simulink model "COSTEP"  (R2024b)
settings: Solver=FixedStepAuto  StartTime=0.0  StopTime=25  FixedStep=1/3600  RelTol=1e-3
model workspace (MAT data in the model file):
  AD : Simulink.Parameter (value not decoded)
  AG : Simulink.Parameter (value not decoded)
  AH : Simulink.Parameter (value not decoded)
  AV : Simulink.Parameter (value not decoded)
  AVP : Simulink.Parameter (value not decoded)
  BCHL : Simulink.Parameter (value not decoded)
  BCHV : Simulink.Parameter (value not decoded)
  BD : Simulink.Parameter (value not decoded)
  BDIST : Simulink.Parameter (value not decoded)
  BG : Simulink.Parameter (value not decoded)
  BH : Simulink.Parameter (value not decoded)
  BVP : Simulink.Parameter (value not decoded)
  CD : Simulink.Parameter (value not decoded)
  CDIST : Simulink.Parameter (value not decoded)
  CG : Simulink.Parameter (value not decoded)
  CH : Simulink.Parameter (value not decoded)
  CVP : Simulink.Parameter (value not decoded)
  DDIST : Simulink.Parameter (value not decoded)
  DIST_CONST : Simulink.Parameter (value not decoded)
  ISV : Simulink.Parameter (value not decoded)
  TLAST : Simulink.Parameter (value not decoded)
  TNEXT : Simulink.Parameter (value not decoded)
  XMW : Simulink.Parameter (value not decoded)
  XNS : Simulink.Parameter (value not decoded)
  XNS2 : Simulink.Parameter (value not decoded)
  XNS3 : Simulink.Parameter (value not decoded)
  XNSADD : Simulink.Parameter (value not decoded)
  XNSE : Simulink.Parameter (value not decoded)
symbols that are objects in the model workspace (value not decoded): AD, AG, AH, AV, AVP, BD, BG, BH, BVP, CD, CG, CH, CVP, XMW, XNS, XNS2, XNS3, XNSE
undefined symbols (not defined in the file or in its folder): magnitude, msgbox, SETPT, XMEAS, XMV
libraries: mylib x381, dspindex x31
(part 10 of 12)

== system COSTEP/Stream Measurements/Subsystem6/Condenser product stream/Subsystem/TST(8a) Temperature of Stream °C  ==
  HST : Inport  PortDimensions=1
  XLR : Inport  Port=2  PortDimensions=8
  ITY : Inport  Port=3
  "AG(I) Coefficient A to determine Enthalpy MBtu/lb·°F " : Constant  Value=AG
  "AH(I) Coefficient A to determine Enthalpy MBtu/lb·°F " : Constant  Value=AH
  AV(I) Coefficient AV to determine Enthalpy MBtu/lb : Constant  Value=AV
  BG(I) Coefficient B to determine Enthalpy MBtu/lb·°F² : Constant  Value=BG
  BH(I) Coefficient B to determine Enthalpy MBtu/lb·°F² : Constant  Value=BH
  CG(I) Coefficient C to determine Enthalpy MBtu/lb·°F³ : Constant  Value=CG
  CH(I) Coefficient C to determine Enthalpy MBtu/lb·°F³ : Constant  Value=CH
  Delay : Delay  DelayLength=1  InitialCondition=0
  MATLAB Function : MATLAB Function  TreatAsAtomicUnit=on
  "XMW(I) Molecular weight of components lb/lb-mol " : Constant  Value=XMW
  TST(8a) : Outport  PortDimensions=1  VectorParamsAs1DForOutWhenUnconnected=off
  wires:
  MATLAB Function/1(TST) -> Delay/1, TST(8a)/1
  Delay/1 -> MATLAB Function/12("TST ")
  "AG(I) Coefficient A to determine Enthalpy MBtu/lb·°F "/1 -> MATLAB Function/4(AG)
  AV(I) Coefficient AV to determine Enthalpy MBtu/lb/1 -> MATLAB Function/7(AV)
  HST/1 -> MATLAB Function/10(HST)
  CH(I) Coefficient C to determine Enthalpy MBtu/lb·°F³/1 -> MATLAB Function/3(CH)
  ITY/1 -> MATLAB Function/11(ITY)
  "XMW(I) Molecular weight of components lb/lb-mol "/1 -> MATLAB Function/8(XMW)
  XLR/1 -> MATLAB Function/9(XLR)
  "AH(I) Coefficient A to determine Enthalpy MBtu/lb·°F "/1 -> MATLAB Function/1(AH)
  CG(I) Coefficient C to determine Enthalpy MBtu/lb·°F³/1 -> MATLAB Function/6(CG)
  BH(I) Coefficient B to determine Enthalpy MBtu/lb·°F²/1 -> MATLAB Function/2(BH)
  BG(I) Coefficient B to determine Enthalpy MBtu/lb·°F²/1 -> MATLAB Function/5(BG)

== system COSTEP/Stream Measurements/Subsystem6/D feed stream/Composition measurement mol%/Subsystem ==
  XST : Inport
  XMNSE : Inport  Port=2
  Bus Selector : BusSelector  OutputSignals=XMNSEB,XMNSED
  Process Noise I=23-1 : mylib/Process Noise I=23-36  SystemSampleTime=-1  VariantActivationTime=update diagram  AllowFlexibleInterface=on  Latency=0  AutoFrameSizeCalculation=off
  Process Noise I=23-3 : mylib/Process Noise I=23-36  SystemSampleTime=-1  VariantActivationTime=update diagram  AllowFlexibleInterface=on  Latency=0  AutoFrameSizeCalculation=off
  Subsystem : Subsystem
  SMEASXB(2) : Outport  VectorParamsAs1DForOutWhenUnconnected=off
  SMEASXD(2) : Outport  Port=2  VectorParamsAs1DForOutWhenUnconnected=off
  wires:
  Process Noise I=23-1/1 -> SMEASXB(2)/1
  Bus Selector/1 -> Process Noise I=23-1/2  "<XMNSEB>"
  Process Noise I=23-3/1 -> SMEASXD(2)/1
  Bus Selector/2 -> Process Noise I=23-3/2  "<XMNSED>"
  XST/1 -> Subsystem/1(XST)
  Subsystem/1(XCMPB) -> Process Noise I=23-1/1
  Subsystem/2(XCMPD) -> Process Noise I=23-3/1
  XMNSE/1 -> Bus Selector/1

== system COSTEP/Stream Measurements/Subsystem6/E feed stream/Composition measurement mol%/Subsystem ==
  XST : Inport
  XMNSE : Inport  Port=2
  Bus Selector : BusSelector  OutputSignals=XMNSEE,XMNSEF
  Process Noise I=23-4 : mylib/Process Noise I=23-36  SystemSampleTime=-1  VariantActivationTime=update diagram  AllowFlexibleInterface=on  Latency=0  AutoFrameSizeCalculation=off
  Process Noise I=23-5 : mylib/Process Noise I=23-36  SystemSampleTime=-1  VariantActivationTime=update diagram  AllowFlexibleInterface=on  Latency=0  AutoFrameSizeCalculation=off
  Subsystem : Subsystem
  SMEASXE(3) : Outport  VectorParamsAs1DForOutWhenUnconnected=off
  SMEASXF(3) : Outport  Port=2  VectorParamsAs1DForOutWhenUnconnected=off
  wires:
  Process Noise I=23-4/1 -> SMEASXE(3)/1
  Process Noise I=23-5/1 -> SMEASXF(3)/1
  Bus Selector/2 -> Process Noise I=23-5/2  "<XMNSEF>"
  Bus Selector/1 -> Process Noise I=23-4/2  "<XMNSEE>"
  XST/1 -> Subsystem/1(XST)
  Subsystem/1("XCMPE ") -> Process Noise I=23-4/1
  Subsystem/2("XCMPF ") -> Process Noise I=23-5/1
  XMNSE/1 -> Bus Selector/1

== system COSTEP/Stream Measurements/Subsystem6/Product stream/Composition measurement mol%/Subsystem ==
  XST : Inport
  XMNSE : Inport  Port=2
  Bus Selector : BusSelector  OutputSignals=XMNSEA,XMNSEB,XMNSEC
  Process Noise I=23-1 : mylib/Process Noise I=23-36  SystemSampleTime=-1  VariantActivationTime=update diagram  AllowFlexibleInterface=on  Latency=0  AutoFrameSizeCalculation=off
  Process Noise I=23-2 : mylib/Process Noise I=23-36  SystemSampleTime=-1  VariantActivationTime=update diagram  AllowFlexibleInterface=on  Latency=0  AutoFrameSizeCalculation=off
  Process Noise I=23-36 : mylib/Process Noise I=23-36  SystemSampleTime=-1  VariantActivationTime=update diagram  AllowFlexibleInterface=on  Latency=0  AutoFrameSizeCalculation=off
  Subsystem : Subsystem
  SMEASXA : Outport  VectorParamsAs1DForOutWhenUnconnected=off
  SMEASXB : Outport  Port=2  VectorParamsAs1DForOutWhenUnconnected=off
  SMEASXC : Outport  Port=3  VectorParamsAs1DForOutWhenUnconnected=off
  wires:
  Process Noise I=23-36/1 -> SMEASXA/1
  Process Noise I=23-1/1 -> SMEASXB/1
  Bus Selector/2 -> Process Noise I=23-1/2  "<XMNSEB>"
  Process Noise I=23-2/1 -> SMEASXC/1
  Bus Selector/3 -> Process Noise I=23-2/2  "<XMNSEC>"
  Bus Selector/1 -> Process Noise I=23-36/2  "<XMNSEA>"
  XST/1 -> Subsystem/1(XST)
  Subsystem/1(XCMPA) -> Process Noise I=23-36/1
  Subsystem/2(XCMPB) -> Process Noise I=23-1/1
  Subsystem/3(XCMPC) -> Process Noise I=23-2/1
  XMNSE/1 -> Bus Selector/1

== system COSTEP/Stream Measurements/Subsystem6/Product stream/Composition measurement mol%/Subsystem1 ==
  XST : Inport
  XMNSE3 : Inport  Port=2
  Bus Selector : BusSelector  OutputSignals=XMNSED,XMNSEE,XMNSEF,XMNSEG,XMNSEH
  Process Noise I=37-{1..4,41} (5 alike) : mylib/Process Noise I=37-41  SystemSampleTime=-1  VariantActivationTime=update diagram  AllowFlexibleInterface=on  Latency=0  AutoFrameSizeCalculation=off
  Subsystem : Subsystem
  SMEASXD : Outport  VectorParamsAs1DForOutWhenUnconnected=off
  SMEASXE : Outport  Port=2  VectorParamsAs1DForOutWhenUnconnected=off
  SMEASXF : Outport  Port=3  VectorParamsAs1DForOutWhenUnconnected=off
  SMEASXG : Outport  Port=4  VectorParamsAs1DForOutWhenUnconnected=off
  SMEASXH : Outport  Port=5  VectorParamsAs1DForOutWhenUnconnected=off
  wires:
  Process Noise I=37-41/1 -> SMEASXD/1
  Bus Selector/1 -> Process Noise I=37-41/2  "<XMNSED>"
  Process Noise I=37-1/1 -> SMEASXE/1
  Bus Selector/2 -> Process Noise I=37-1/2  "<XMNSEE>"
  Process Noise I=37-2/1 -> SMEASXF/1
  Bus Selector/3 -> Process Noise I=37-2/2  "<XMNSEF>"
  Process Noise I=37-3/1 -> SMEASXG/1
  Bus Selector/4 -> Process Noise I=37-3/2  "<XMNSEG>"
  Process Noise I=37-4/1 -> SMEASXH/1
  Bus Selector/5 -> Process Noise I=37-4/2  "<XMNSEH>"
  XST/1 -> Subsystem/1(XST)
  Subsystem/1(XCMPD) -> Process Noise I=37-41/1
  Subsystem/2("XCMPE ") -> Process Noise I=37-1/1
  Subsystem/3("XCMPF ") -> Process Noise I=37-2/1
  Subsystem/4(XCMPG) -> Process Noise I=37-3/1
  Subsystem/5("XCMPH ") -> Process Noise I=37-4/1
  XMNSE3/1 -> Bus Selector/1

== system COSTEP/Stream Measurements/Subsystem6/Product stream/Flow measurement in kg//h/XMWS Molecular weight of Stream lb//lb-mol ==
  XST : Inport
  Product : Product
  Sum of Elements : Sum  Inputs=+
  "XMW(I) Molecular weight of components lb/lb-mol " : Constant  Value=XMW
  XMWS : Outport  VectorParamsAs1DForOutWhenUnconnected=off
  wires:
  Sum of Elements/1 -> XMWS/1
  Product/1 -> Sum of Elements/1
  XST/1 -> Product/1
  "XMW(I) Molecular weight of components lb/lb-mol "/1 -> Product/2

== system COSTEP/Stream Measurements/Subsystem6/Purge stream/Flow measurement in kg//h/XMWS Molecular weight of Stream lb//lb-mol ==
  XST : Inport
  Product : Product
  Sum of Elements : Sum  Inputs=+
  "XMW(I) Molecular weight of components lb/lb-mol " : Constant  Value=XMW
  XMWS : Outport  VectorParamsAs1DForOutWhenUnconnected=off
  wires:
  Sum of Elements/1 -> XMWS/1
  Product/1 -> Sum of Elements/1
  XST/1 -> Product/1
  "XMW(I) Molecular weight of components lb/lb-mol "/1 -> Product/2

== system COSTEP/Stream Measurements/Subsystem6/Reactor feed stream/Composition measurement mol%/Subsystem ==
  XST : Inport
  XMNSE : Inport  Port=2
  XMEAS : Inport  Port=3
  Bus Selector : BusSelector  OutputSignals=XMNSEG,XMNSEH
  Bus Selector1 : BusSelector  OutputSignals=XMEAS(23),XMEAS(24),XMEAS(25),XMEAS(26),XMEAS(27),XMEAS(28)
  Process Noise I=23-6 : mylib/Process Noise I=23-36  SystemSampleTime=-1  VariantActivationTime=update diagram  AllowFlexibleInterface=on  Latency=0  AutoFrameSizeCalculation=off
  Process Noise I=23-7 : mylib/Process Noise I=23-36  SystemSampleTime=-1  VariantActivationTime=update diagram  AllowFlexibleInterface=on  Latency=0  AutoFrameSizeCalculation=off
  Subsystem : Subsystem
  SMEASXA : Outport  VectorParamsAs1DForOutWhenUnconnected=off
  SMEASXB : Outport  Port=2  VectorParamsAs1DForOutWhenUnconnected=off
  SMEASXC : Outport  Port=3  VectorParamsAs1DForOutWhenUnconnected=off
  SMEASXD : Outport  Port=4  VectorParamsAs1DForOutWhenUnconnected=off
  SMEASXE : Outport  Port=5  VectorParamsAs1DForOutWhenUnconnected=off
  SMEASXF : Outport  Port=6  VectorParamsAs1DForOutWhenUnconnected=off
  SMEASXG : Outport  Port=7  VectorParamsAs1DForOutWhenUnconnected=off
  SMEASXH : Outport  Port=8  VectorParamsAs1DForOutWhenUnconnected=off
  wires:
  Bus Selector1/1 -> SMEASXA/1  "<XMEAS(23)>"
  Bus Selector1/2 -> SMEASXB/1  "<XMEAS(24)>"
  Bus Selector1/3 -> SMEASXC/1  "<XMEAS(25)>"
  Bus Selector1/4 -> SMEASXD/1  "<XMEAS(26)>"
  Bus Selector1/5 -> SMEASXE/1  "<XMEAS(27)>"
  Bus Selector1/6 -> SMEASXF/1  "<XMEAS(28)>"
  Process Noise I=23-6/1 -> SMEASXG/1
  Process Noise I=23-7/1 -> SMEASXH/1
  Bus Selector/1 -> Process Noise I=23-6/2  "<XMNSEG>"
  Bus Selector/2 -> Process Noise I=23-7/2  "<XMNSEH>"
  XST/1 -> Subsystem/1(XST)
  Subsystem/1(XCMPG) -> Process Noise I=23-6/1
  Subsystem/2("XCMPH ") -> Process Noise I=23-7/1
  XMNSE/1 -> Bus Selector/1
  XMEAS/1 -> Bus Selector1/1

== system COSTEP/Stream Measurements/Subsystem6/Reactor feed stream/Flow measurement in kg//h/XMWS Molecular weight of Stream lb//lb-mol ==
  XST : Inport
  Product : Product
  Sum of Elements : Sum  Inputs=+
  "XMW(I) Molecular weight of components lb/lb-mol " : Constant  Value=XMW
  XMWS : Outport  VectorParamsAs1DForOutWhenUnconnected=off
  wires:
  Sum of Elements/1 -> XMWS/1
  Product/1 -> Sum of Elements/1
  XST/1 -> Product/1
  "XMW(I) Molecular weight of components lb/lb-mol "/1 -> Product/2

== system COSTEP/Stream Measurements/Subsystem6/Reactor product stream/Composition measurement mol%/Subsystem ==
  XST : Inport
  XMNSE : Inport  Port=2
  Bus Selector : BusSelector  OutputSignals=XMNSEA,XMNSEB,XMNSEC,XMNSED,XMNSEE,XMNSEF,XMNSEG,XMNSEH
  Process Noise I=23-{1..7,36} (8 alike) : mylib/Process Noise I=23-36  SystemSampleTime=-1  VariantActivationTime=update diagram  AllowFlexibleInterface=on  Latency=0  AutoFrameSizeCalculation=off
  Subsystem : Subsystem
  SMEASXA(7) : Outport  VectorParamsAs1DForOutWhenUnconnected=off
  SMEASXB(7) : Outport  Port=2  VectorParamsAs1DForOutWhenUnconnected=off
  SMEASXC(7) : Outport  Port=3  VectorParamsAs1DForOutWhenUnconnected=off
  SMEASXD(7) : Outport  Port=4  VectorParamsAs1DForOutWhenUnconnected=off
  SMEASXE(7) : Outport  Port=5  VectorParamsAs1DForOutWhenUnconnected=off
  SMEASXF(7) : Outport  Port=6  VectorParamsAs1DForOutWhenUnconnected=off
  SMEASXG(7) : Outport  Port=7  VectorParamsAs1DForOutWhenUnconnected=off
  SMEASXH(7) : Outport  Port=8  VectorParamsAs1DForOutWhenUnconnected=off
  wires:
  Process Noise I=23-36/1 -> SMEASXA(7)/1
  Process Noise I=23-1/1 -> SMEASXB(7)/1
  Bus Selector/2 -> Process Noise I=23-1/2  "<XMNSEB>"
  Process Noise I=23-2/1 -> SMEASXC(7)/1
  Process Noise I=23-3/1 -> SMEASXD(7)/1
  Process Noise I=23-4/1 -> SMEASXE(7)/1
  Process Noise I=23-5/1 -> SMEASXF(7)/1
  Process Noise I=23-6/1 -> SMEASXG(7)/1
  Process Noise I=23-7/1 -> SMEASXH(7)/1
  Bus Selector/7 -> Process Noise I=23-6/2  "<XMNSEG>"
  Bus Selector/8 -> Process Noise I=23-7/2  "<XMNSEH>"
  Bus Selector/6 -> Process Noise I=23-5/2  "<XMNSEF>"
  Bus Selector/5 -> Process Noise I=23-4/2  "<XMNSEE>"
  Bus Selector/4 -> Process Noise I=23-3/2  "<XMNSED>"
  Bus Selector/3 -> Process Noise I=23-2/2  "<XMNSEC>"
  Bus Selector/1 -> Process Noise I=23-36/2  "<XMNSEA>"
  XST/1 -> Subsystem/1(XST)
  Subsystem/1(XCMPA) -> Process Noise I=23-36/1
  Subsystem/2(XCMPB) -> Process Noise I=23-1/1
  Subsystem/3(XCMPC) -> Process Noise I=23-2/1
  Subsystem/4(XCMPD) -> Process Noise I=23-3/1
  Subsystem/5("XCMPE ") -> Process Noise I=23-4/1
  Subsystem/6("XCMPF ") -> Process Noise I=23-5/1
  Subsystem/7(XCMPG) -> Process Noise I=23-6/1
  Subsystem/8("XCMPH ") -> Process Noise I=23-7/1
  XMNSE/1 -> Bus Selector/1

== system COSTEP/Stream Measurements/Subsystem6/Reactor product stream/Flow measurement in kg//h/XMWS Molecular weight of Stream lb//lb-mol ==
  XST : Inport
  Product : Product
  Sum of Elements : Sum  Inputs=+
  "XMW(I) Molecular weight of components lb/lb-mol " : Constant  Value=XMW
  XMWS : Outport  VectorParamsAs1DForOutWhenUnconnected=off
  wires:
  Sum of Elements/1 -> XMWS/1
  Product/1 -> Sum of Elements/1
  XST/1 -> Product/1
  "XMW(I) Molecular weight of components lb/lb-mol "/1 -> Product/2

== system COSTEP/Stream Measurements/Subsystem6/Separator product stream/Composition measurement mol%/Subsystem ==
  XST : Inport
  XMNSE : Inport  Port=2
  Bus Selector : BusSelector  OutputSignals=XMNSEA,XMNSEB,XMNSEC,XMNSED,XMNSEE,XMNSEF,XMNSEG,XMNSEH
  Process Noise I=23-{1..7,36} (8 alike) : mylib/Process Noise I=23-36  SystemSampleTime=-1  VariantActivationTime=update diagram  AllowFlexibleInterface=on  Latency=0  AutoFrameSizeCalculation=off
  Subsystem : Subsystem
  SMEASXA : Outport  VectorParamsAs1DForOutWhenUnconnected=off
  SMEASXB : Outport  Port=2  VectorParamsAs1DForOutWhenUnconnected=off
  SMEASXC : Outport  Port=3  VectorParamsAs1DForOutWhenUnconnected=off
  SMEASXD : Outport  Port=4  VectorParamsAs1DForOutWhenUnconnected=off
  SMEASXE : Outport  Port=5  VectorParamsAs1DForOutWhenUnconnected=off
  SMEASXF : Outport  Port=6  VectorParamsAs1DForOutWhenUnconnected=off
  SMEASXG : Outport  Port=7  VectorParamsAs1DForOutWhenUnconnected=off
  SMEASXH : Outport  Port=8  VectorParamsAs1DForOutWhenUnconnected=off
  wires:
  Process Noise I=23-36/1 -> SMEASXA/1
  Process Noise I=23-1/1 -> SMEASXB/1
  Bus Selector/2 -> Process Noise I=23-1/2  "<XMNSEB>"
  Process Noise I=23-2/1 -> SMEASXC/1
  Process Noise I=23-3/1 -> SMEASXD/1
  Process Noise I=23-4/1 -> SMEASXE/1
  Process Noise I=23-5/1 -> SMEASXF/1
  Process Noise I=23-6/1 -> SMEASXG/1
  Process Noise I=23-7/1 -> SMEASXH/1
  Bus Selector/7 -> Process Noise I=23-6/2  "<XMNSEG>"
  Bus Selector/8 -> Process Noise I=23-7/2  "<XMNSEH>"
  Bus Selector/6 -> Process Noise I=23-5/2  "<XMNSEF>"
  Bus Selector/5 -> Process Noise I=23-4/2  "<XMNSEE>"
  Bus Selector/4 -> Process Noise I=23-3/2  "<XMNSED>"
  Bus Selector/3 -> Process Noise I=23-2/2  "<XMNSEC>"
  Bus Selector/1 -> Process Noise I=23-36/2  "<XMNSEA>"
  XST/1 -> Subsystem/1(XST)
  Subsystem/1(XCMPA) -> Process Noise I=23-36/1
  Subsystem/2(XCMPB) -> Process Noise I=23-1/1
  Subsystem/3(XCMPC) -> Process Noise I=23-2/1
  Subsystem/4(XCMPD) -> Process Noise I=23-3/1
  Subsystem/5("XCMPE ") -> Process Noise I=23-4/1
  Subsystem/6("XCMPF ") -> Process Noise I=23-5/1
  Subsystem/7(XCMPG) -> Process Noise I=23-6/1
  Subsystem/8("XCMPH ") -> Process Noise I=23-7/1
  XMNSE/1 -> Bus Selector/1

== system COSTEP/Stream Measurements/Subsystem6/Separator product stream/Flow measurement in kg//h/Subsystem ==
  XST : Inport
  XMEAS : Inport  Port=2
  " " : Constant  Value=35.3145
  "  " : Constant  Value=0.359
  Convert from lb/h to kg/h : Constant  Value=0.454
  Product : Product  Inputs=3
  XMWS Molecular weight of Stream lb/lb-mol : Subsystem
  lb-mol/h : Product  Inputs=**/
  SMEAS F : Outport
  wires:
  lb-mol/h/1 -> Product/2
  " "/1 -> lb-mol/h/2
  XST/1 -> XMWS Molecular weight of Stream lb/lb-mol/1(XST)
  "  "/1 -> lb-mol/h/3
  Product/1 -> SMEAS F/1
  Convert from lb/h to kg/h/1 -> Product/3
  XMWS Molecular weight of Stream lb/lb-mol/1(XMWS) -> Product/1
  XMEAS/1 -> lb-mol/h/1

== system COSTEP/Stream Measurements/Subsystem6/Separator product stream/Flow measurement in kg//h/Subsystem1 ==
  XST : Inport
  XMEAS : Inport  Port=2
  " " : Constant  Value=35.3145
  "  " : Constant  Value=0.359
  Convert from lb/h to kg/h : Constant  Value=0.454
  Product : Product  Inputs=3
  XMWS Molecular weight of Stream lb/lb-mol : Subsystem
  lb-mol/h : Product  Inputs=**/
  SMEAS F : Outport
  wires:
  lb-mol/h/1 -> Product/2
  " "/1 -> lb-mol/h/2
  XST/1 -> XMWS Molecular weight of Stream lb/lb-mol/1(XST)
  "  "/1 -> lb-mol/h/3
  Product/1 -> SMEAS F/1
  Convert from lb/h to kg/h/1 -> Product/3
  XMWS Molecular weight of Stream lb/lb-mol/1(XMWS) -> Product/1
  XMEAS/1 -> lb-mol/h/1

== system COSTEP/Stream Measurements/Subsystem6/Separator recycle stream (after compressor)/Composition measurement mol%/Subsystem ==
  XST : Inport
  XMNSE : Inport  Port=2
  Bus Selector : BusSelector  OutputSignals=XMNSEA,XMNSEB,XMNSEC,XMNSED,XMNSEE,XMNSEF,XMNSEG,XMNSEH
  Process Noise I=23-{1..7,36} (8 alike) : mylib/Process Noise I=23-36  SystemSampleTime=-1  VariantActivationTime=update diagram  AllowFlexibleInterface=on  Latency=0  AutoFrameSizeCalculation=off
  Subsystem : Subsystem
  SMEASXA : Outport  VectorParamsAs1DForOutWhenUnconnected=off
  SMEASXB : Outport  Port=2  VectorParamsAs1DForOutWhenUnconnected=off
  SMEASXC : Outport  Port=3  VectorParamsAs1DForOutWhenUnconnected=off
  SMEASXD : Outport  Port=4  VectorParamsAs1DForOutWhenUnconnected=off
  SMEASXE : Outport  Port=5  VectorParamsAs1DForOutWhenUnconnected=off
  SMEASXF : Outport  Port=6  VectorParamsAs1DForOutWhenUnconnected=off
  SMEASXG : Outport  Port=7  VectorParamsAs1DForOutWhenUnconnected=off
  SMEASXH : Outport  Port=8  VectorParamsAs1DForOutWhenUnconnected=off
  wires:
  Process Noise I=23-36/1 -> SMEASXA/1
  Process Noise I=23-1/1 -> SMEASXB/1
  Bus Selector/2 -> Process Noise I=23-1/2  "<XMNSEB>"
  Process Noise I=23-2/1 -> SMEASXC/1
  Process Noise I=23-3/1 -> SMEASXD/1
  Process Noise I=23-4/1 -> SMEASXE/1
  Process Noise I=23-5/1 -> SMEASXF/1
  Process Noise I=23-6/1 -> SMEASXG/1
  Process Noise I=23-7/1 -> SMEASXH/1
  Bus Selector/7 -> Process Noise I=23-6/2  "<XMNSEG>"
  Bus Selector/8 -> Process Noise I=23-7/2  "<XMNSEH>"
  Bus Selector/6 -> Process Noise I=23-5/2  "<XMNSEF>"
  Bus Selector/5 -> Process Noise I=23-4/2  "<XMNSEE>"
  Bus Selector/4 -> Process Noise I=23-3/2  "<XMNSED>"
  Bus Selector/3 -> Process Noise I=23-2/2  "<XMNSEC>"
  Bus Selector/1 -> Process Noise I=23-36/2  "<XMNSEA>"
  XST/1 -> Subsystem/1(XST)
  Subsystem/1(XCMPA) -> Process Noise I=23-36/1
  Subsystem/2(XCMPB) -> Process Noise I=23-1/1
  Subsystem/3(XCMPC) -> Process Noise I=23-2/1
  Subsystem/4(XCMPD) -> Process Noise I=23-3/1
  Subsystem/5("XCMPE ") -> Process Noise I=23-4/1
  Subsystem/6("XCMPF ") -> Process Noise I=23-5/1
  Subsystem/7(XCMPG) -> Process Noise I=23-6/1
  Subsystem/8("XCMPH ") -> Process Noise I=23-7/1
  XMNSE/1 -> Bus Selector/1

== system COSTEP/Stream Measurements/Subsystem6/Separator recycle stream (after compressor)/Flow measurement in kg//h/XMWS Molecular weight of Stream lb//lb-mol ==
  XST : Inport
  Product : Product
  Sum of Elements : Sum  Inputs=+
  "XMW(I) Molecular weight of components lb/lb-mol " : Constant  Value=XMW
  XMWS : Outport  VectorParamsAs1DForOutWhenUnconnected=off
  wires:
  Sum of Elements/1 -> XMWS/1
  Product/1 -> Sum of Elements/1
  XST/1 -> Product/1
  "XMW(I) Molecular weight of components lb/lb-mol "/1 -> Product/2

== system COSTEP/Stream Measurements/Subsystem6/Separator recycle stream (after compressor)/Temperature measurement in C/TST(9) Temperature of Stream °C  ==
  HST : Inport  PortDimensions=1
  XLR : Inport  Port=2  PortDimensions=8
  ITY : Inport  Port=3
  "AG(I) Coefficient A to determine Enthalpy MBtu/lb·°F " : Constant  Value=AG
  "AH(I) Coefficient A to determine Enthalpy MBtu/lb·°F " : Constant  Value=AH
  AV(I) Coefficient AV to determine Enthalpy MBtu/lb : Constant  Value=AV
  BG(I) Coefficient B to determine Enthalpy MBtu/lb·°F² : Constant  Value=BG
  BH(I) Coefficient B to determine Enthalpy MBtu/lb·°F² : Constant  Value=BH
  CG(I) Coefficient C to determine Enthalpy MBtu/lb·°F³ : Constant  Value=CG
  CH(I) Coefficient C to determine Enthalpy MBtu/lb·°F³ : Constant  Value=CH
  Delay : Delay  DelayLength=1  InitialCondition=0
  MATLAB Function : MATLAB Function  TreatAsAtomicUnit=on
  "XMW(I) Molecular weight of components lb/lb-mol " : Constant  Value=XMW
  TST(9) : Outport  PortDimensions=1  VectorParamsAs1DForOutWhenUnconnected=off
  wires:
  MATLAB Function/1(TST) -> Delay/1, TST(9)/1
  Delay/1 -> MATLAB Function/12("TST ")
  "AG(I) Coefficient A to determine Enthalpy MBtu/lb·°F "/1 -> MATLAB Function/4(AG)
  AV(I) Coefficient AV to determine Enthalpy MBtu/lb/1 -> MATLAB Function/7(AV)
  HST/1 -> MATLAB Function/10(HST)
  CH(I) Coefficient C to determine Enthalpy MBtu/lb·°F³/1 -> MATLAB Function/3(CH)
  ITY/1 -> MATLAB Function/11(ITY)
  "XMW(I) Molecular weight of components lb/lb-mol "/1 -> MATLAB Function/8(XMW)
  XLR/1 -> MATLAB Function/9(XLR)
  "AH(I) Coefficient A to determine Enthalpy MBtu/lb·°F "/1 -> MATLAB Function/1(AH)
  CG(I) Coefficient C to determine Enthalpy MBtu/lb·°F³/1 -> MATLAB Function/6(CG)
  BH(I) Coefficient B to determine Enthalpy MBtu/lb·°F²/1 -> MATLAB Function/2(BH)
  BG(I) Coefficient B to determine Enthalpy MBtu/lb·°F²/1 -> MATLAB Function/5(BG)

== system COSTEP/Stream Measurements/Subsystem6/Separator recycle stream (before compressor)/Composition measurement mol%/Subsystem ==
  XST : Inport
  XMNSE : Inport  Port=2
  Bus Selector : BusSelector  OutputSignals=XMNSEA,XMNSEB,XMNSEC,XMNSED,XMNSEE,XMNSEF,XMNSEG,XMNSEH
  Process Noise I=23-{1..7,36} (8 alike) : mylib/Process Noise I=23-36  SystemSampleTime=-1  VariantActivationTime=update diagram  AllowFlexibleInterface=on  Latency=0  AutoFrameSizeCalculation=off
  Subsystem : Subsystem
  SMEASXA : Outport  VectorParamsAs1DForOutWhenUnconnected=off
  SMEASXB : Outport  Port=2  VectorParamsAs1DForOutWhenUnconnected=off
  SMEASXC : Outport  Port=3  VectorParamsAs1DForOutWhenUnconnected=off
  SMEASXD : Outport  Port=4  VectorParamsAs1DForOutWhenUnconnected=off
  SMEASXE : Outport  Port=5  VectorParamsAs1DForOutWhenUnconnected=off
  SMEASXF : Outport  Port=6  VectorParamsAs1DForOutWhenUnconnected=off
  SMEASXG : Outport  Port=7  VectorParamsAs1DForOutWhenUnconnected=off
  SMEASXH : Outport  Port=8  VectorParamsAs1DForOutWhenUnconnected=off
  wires:
  Process Noise I=23-36/1 -> SMEASXA/1
  Process Noise I=23-1/1 -> SMEASXB/1
  Bus Selector/2 -> Process Noise I=23-1/2  "<XMNSEB>"
  Process Noise I=23-2/1 -> SMEASXC/1
  Process Noise I=23-3/1 -> SMEASXD/1
  Process Noise I=23-4/1 -> SMEASXE/1
  Process Noise I=23-5/1 -> SMEASXF/1
  Process Noise I=23-6/1 -> SMEASXG/1
  Process Noise I=23-7/1 -> SMEASXH/1
  Bus Selector/7 -> Process Noise I=23-6/2  "<XMNSEG>"
  Bus Selector/8 -> Process Noise I=23-7/2  "<XMNSEH>"
  Bus Selector/6 -> Process Noise I=23-5/2  "<XMNSEF>"
  Bus Selector/5 -> Process Noise I=23-4/2  "<XMNSEE>"
  Bus Selector/4 -> Process Noise I=23-3/2  "<XMNSED>"
  Bus Selector/3 -> Process Noise I=23-2/2  "<XMNSEC>"
  Bus Selector/1 -> Process Noise I=23-36/2  "<XMNSEA>"
  XST/1 -> Subsystem/1(XST)
  Subsystem/1(XCMPA) -> Process Noise I=23-36/1
  Subsystem/2(XCMPB) -> Process Noise I=23-1/1
  Subsystem/3(XCMPC) -> Process Noise I=23-2/1
  Subsystem/4(XCMPD) -> Process Noise I=23-3/1
  Subsystem/5("XCMPE ") -> Process Noise I=23-4/1
  Subsystem/6("XCMPF ") -> Process Noise I=23-5/1
  Subsystem/7(XCMPG) -> Process Noise I=23-6/1
  Subsystem/8("XCMPH ") -> Process Noise I=23-7/1
  XMNSE/1 -> Bus Selector/1

== system COSTEP/Stream Measurements/Subsystem6/Separator recycle stream (before compressor)/Flow measurement in kg//h/XMWS Molecular weight of Stream lb//lb-mol ==
  XST : Inport
  Product : Product
  Sum of Elements : Sum  Inputs=+
  "XMW(I) Molecular weight of components lb/lb-mol " : Constant  Value=XMW
  XMWS : Outport  VectorParamsAs1DForOutWhenUnconnected=off
  wires:
  Sum of Elements/1 -> XMWS/1
  Product/1 -> Sum of Elements/1
  XST/1 -> Product/1
  "XMW(I) Molecular weight of components lb/lb-mol "/1 -> Product/2

== system COSTEP/Stream Measurements/Subsystem6/Separator underflow stream/Composition measurement mol%/Subsystem ==
  XST : Inport
  XMNSE : Inport  Port=2
  Bus Selector : BusSelector  OutputSignals=XMNSED,XMNSEE,XMNSEF,XMNSEG,XMNSEH
  Process Noise I=23-{3..7} (5 alike) : mylib/Process Noise I=23-36  SystemSampleTime=-1  VariantActivationTime=update diagram  AllowFlexibleInterface=on  Latency=0  AutoFrameSizeCalculation=off
  Subsystem : Subsystem
  SMEASXD : Outport  VectorParamsAs1DForOutWhenUnconnected=off
  SMEASXE : Outport  Port=2  VectorParamsAs1DForOutWhenUnconnected=off
  SMEASXF : Outport  Port=3  VectorParamsAs1DForOutWhenUnconnected=off
  SMEASXG : Outport  Port=4  VectorParamsAs1DForOutWhenUnconnected=off
  SMEASXH : Outport  Port=5  VectorParamsAs1DForOutWhenUnconnected=off
  wires:
  Process Noise I=23-3/1 -> SMEASXD/1
  Process Noise I=23-4/1 -> SMEASXE/1
  Process Noise I=23-5/1 -> SMEASXF/1
  Process Noise I=23-6/1 -> SMEASXG/1
  Process Noise I=23-7/1 -> SMEASXH/1
  Bus Selector/4 -> Process Noise I=23-6/2  "<XMNSEG>"
  Bus Selector/5 -> Process Noise I=23-7/2  "<XMNSEH>"
  Bus Selector/3 -> Process Noise I=23-5/2  "<XMNSEF>"
  Bus Selector/2 -> Process Noise I=23-4/2  "<XMNSEE>"
  Bus Selector/1 -> Process Noise I=23-3/2  "<XMNSED>"
  XST/1 -> Subsystem/1(XST)
  Subsystem/1(XCMPD) -> Process Noise I=23-3/1
  Subsystem/2("XCMPE ") -> Process Noise I=23-4/1
  Subsystem/3("XCMPF ") -> Process Noise I=23-5/1
  Subsystem/4(XCMPG) -> Process Noise I=23-6/1
  Subsystem/5("XCMPH ") -> Process Noise I=23-7/1
  XMNSE/1 -> Bus Selector/1

== system COSTEP/Stream Measurements/Subsystem6/Separator underflow stream/Flow measurement in kg//h/XMWS Molecular weight of Stream lb//lb-mol ==
  XST : Inport
  Product : Product
  Sum of Elements : Sum  Inputs=+
  "XMW(I) Molecular weight of components lb/lb-mol " : Constant  Value=XMW
  XMWS : Outport  VectorParamsAs1DForOutWhenUnconnected=off
  wires:
  Sum of Elements/1 -> XMWS/1
  Product/1 -> Sum of Elements/1
  XST/1 -> Product/1
  "XMW(I) Molecular weight of components lb/lb-mol "/1 -> Product/2

== system COSTEP/Stream Measurements/Subsystem6/Stripper recycle stream/Composition measurement mol%/Subsystem ==
  XST : Inport
  XMNSE : Inport  Port=2
  Bus Selector : BusSelector  OutputSignals=XMNSEA,XMNSEB,XMNSEC,XMNSED,XMNSEE,XMNSEF,XMNSEG,XMNSEH
  Process Noise I=23-{1..7,36} (8 alike) : mylib/Process Noise I=23-36  SystemSampleTime=-1  VariantActivationTime=update diagram  AllowFlexibleInterface=on  Latency=0  AutoFrameSizeCalculation=off
  Subsystem : Subsystem
  SMEASXA : Outport  VectorParamsAs1DForOutWhenUnconnected=off
  SMEASXB : Outport  Port=2  VectorParamsAs1DForOutWhenUnconnected=off
  SMEASXC : Outport  Port=3  VectorParamsAs1DForOutWhenUnconnected=off
  SMEASXD : Outport  Port=4  VectorParamsAs1DForOutWhenUnconnected=off
  SMEASXE : Outport  Port=5  VectorParamsAs1DForOutWhenUnconnected=off
  SMEASXF : Outport  Port=6  VectorParamsAs1DForOutWhenUnconnected=off
  SMEASXG : Outport  Port=7  VectorParamsAs1DForOutWhenUnconnected=off
  SMEASXH : Outport  Port=8  VectorParamsAs1DForOutWhenUnconnected=off
  wires:
  Process Noise I=23-36/1 -> SMEASXA/1
  Process Noise I=23-1/1 -> SMEASXB/1
  Bus Selector/2 -> Process Noise I=23-1/2  "<XMNSEB>"
  Process Noise I=23-2/1 -> SMEASXC/1
  Process Noise I=23-3/1 -> SMEASXD/1
  Process Noise I=23-4/1 -> SMEASXE/1
  Process Noise I=23-5/1 -> SMEASXF/1
  Process Noise I=23-6/1 -> SMEASXG/1
  Process Noise I=23-7/1 -> SMEASXH/1
  Bus Selector/7 -> Process Noise I=23-6/2  "<XMNSEG>"
  Bus Selector/8 -> Process Noise I=23-7/2  "<XMNSEH>"
  Bus Selector/6 -> Process Noise I=23-5/2  "<XMNSEF>"
  Bus Selector/5 -> Process Noise I=23-4/2  "<XMNSEE>"
  Bus Selector/4 -> Process Noise I=23-3/2  "<XMNSED>"
  Bus Selector/3 -> Process Noise I=23-2/2  "<XMNSEC>"
  Bus Selector/1 -> Process Noise I=23-36/2  "<XMNSEA>"
  XST/1 -> Subsystem/1(XST)
  Subsystem/1(XCMPA) -> Process Noise I=23-36/1
  Subsystem/2(XCMPB) -> Process Noise I=23-1/1
  Subsystem/3(XCMPC) -> Process Noise I=23-2/1
  Subsystem/4(XCMPD) -> Process Noise I=23-3/1
  Subsystem/5("XCMPE ") -> Process Noise I=23-4/1
  Subsystem/6("XCMPF ") -> Process Noise I=23-5/1
  Subsystem/7(XCMPG) -> Process Noise I=23-6/1
  Subsystem/8("XCMPH ") -> Process Noise I=23-7/1
  XMNSE/1 -> Bus Selector/1

== system COSTEP/Stream Measurements/Subsystem6/Stripper recycle stream/Flow measurement in kg//h/XMWS Molecular weight of Stream lb//lb-mol ==
  XST : Inport
  Product : Product
  Sum of Elements : Sum  Inputs=+
  "XMW(I) Molecular weight of components lb/lb-mol " : Constant  Value=XMW
  XMWS : Outport  VectorParamsAs1DForOutWhenUnconnected=off
  wires:
  Sum of Elements/1 -> XMWS/1
  Product/1 -> Sum of Elements/1
  XST/1 -> Product/1
  "XMW(I) Molecular weight of components lb/lb-mol "/1 -> Product/2

== system COSTEP/Control Mode/Braatz/ /CONTROL 14/PI Control Setpoint Velocity form/Subsystem ==
  Setpoint : Inport
  Measurement : Inport  Port=2
  Controller Gain : Gain  Gain=Kc  SaturateOnIntegerOverflow=on  OutDataTypeStr=Inherit: Same as input  ParamDataTypeStr=Inherit: Same as input
  Error : ZeroOrderHold  SampleTime=Ts
  Error old : UnitDelay  SampleTime=Ts
  Gain : Gain  Gain=100/HS
  Gain1 : Gain  Gain=Ts/Ti  SaturateOnIntegerOverflow=on  OutDataTypeStr=Inherit: Same as input  ParamDataTypeStr=Inherit: Same as input
  Sum : Sum  Inputs=|+-  SaturateOnIntegerOverflow=on
  Sum1 : Sum  Inputs=++-  SaturateOnIntegerOverflow=on
  Delta Output : Outport
  wires:
  Measurement/1 -> Sum/2
  Controller Gain/1 -> Delta Output/1
  Gain1/1 -> Sum1/2
  Setpoint/1 -> Sum/1
  Error old/1 -> Sum1/3
  Sum1/1 -> Controller Gain/1
  Error/1 -> Sum1/1, Error old/1, Gain1/1
  Gain/1 -> Error/1
  Sum/1 -> Gain/1

== system COSTEP/Control Mode/Braatz/ 10/CONTROL 6/P Control Velocity form/Pressure limits ==
  "XMV(6) " : Inport
  XMEAS : Inport  Port=2
  Abs : Abs  SaturateOnIntegerOverflow=off
  Bus Selector : BusSelector  OutputSignals=signal3.XMEAS(13)
  Constant : Constant  Value=100
  Constant1 : Constant  Value=0
  If : If  IfExpression=u1 >= 2950  ElseIfExpressions=u1 <= 2300
  If Action Subsystem : Subsystem  TreatAsAtomicUnit=on
  If Action Subsystem1 : Subsystem  TreatAsAtomicUnit=on
  If Action Subsystem2 : Subsystem  TreatAsAtomicUnit=on
  Merge : Merge  Inputs=3
  Valve Opening Limits : Saturate  UpperLimit=100  LowerLimit=0
  XMV(6) : Outport  VectorParamsAs1DForOutWhenUnconnected=off
  wires:
  If/1 -> If Action Subsystem/Action
  Constant1/1 -> If Action Subsystem1/1(In1)
  Merge/1 -> Abs/1
  If/3 -> If Action Subsystem2/Action
  Constant/1 -> If Action Subsystem/1(In1)
  Bus Selector/1 -> If/1  "<XMEAS(13)>"
  If Action Subsystem2/1(Out1) -> Merge/3
  If Action Subsystem1/1(Out1) -> Merge/2
  XMEAS/1 -> Bus Selector/1
  If/2 -> If Action Subsystem1/Action
  If Action Subsystem/1(Out1) -> Merge/1
  "XMV(6) "/1 -> If Action Subsystem2/1(In1)
  Abs/1 -> Valve Opening Limits/1
  Valve Opening Limits/1 -> XMV(6)/1

== system COSTEP/Control Mode/Braatz/ 10/CONTROL 6/P Control Velocity form/Subsystem ==
  Setpoint : Inport
  Measurement : Inport  Port=2
  Controller Gain : Gain  Gain=Kc  SaturateOnIntegerOverflow=on  OutDataTypeStr=Inherit: Same as input  ParamDataTypeStr=Inherit: Same as input
  Error : ZeroOrderHold  SampleTime=Ts
  Error old : UnitDelay  SampleTime=Ts
  Gain : Gain  Gain=100/H
  Sum : Sum  Inputs=|+-  SaturateOnIntegerOverflow=on
  Sum1 : Sum  Inputs=+-  SaturateOnIntegerOverflow=on
  Delta Output : Outport
  wires:
  Gain/1 -> Error/1
  Sum/1 -> Gain/1
  Error/1 -> Error old/1, Sum1/1
  Sum1/1 -> Controller Gain/1
  Error old/1 -> Sum1/2
  Setpoint/1 -> Sum/1
  Controller Gain/1 -> Delta Output/1
  Measurement/1 -> Sum/2

== system COSTEP/Random number generator/Stream Measurements SMEAS Gas analysis1/If Action Subsystem3/Subsystem/Stream 1/Subsystem ==
  G : Inport
  TESUB6 XMNSEA : Subsystem
  TESUB6 XMNSEB : Subsystem
  TESUB6 XMNSEC : Subsystem
  TESUB6 XMNSED : Subsystem
  TESUB6 XMNSEE : Subsystem
  TESUB6 XMNSEF : Subsystem
  TESUB6 XMNSEG : Subsystem
  TESUB6 XMNSEH : Subsystem
  XMNSEA : Outport  VectorParamsAs1DForOutWhenUnconnected=off
  XMNSEB : Outport  Port=2  VectorParamsAs1DForOutWhenUnconnected=off
  XMNSEC : Outport  Port=3  VectorParamsAs1DForOutWhenUnconnected=off
  XMNSED : Outport  Port=4  VectorParamsAs1DForOutWhenUnconnected=off
  XMNSEE : Outport  Port=5  VectorParamsAs1DForOutWhenUnconnected=off
  XMNSEF : Outport  Port=6  VectorParamsAs1DForOutWhenUnconnected=off
  XMNSEG : Outport  Port=7  VectorParamsAs1DForOutWhenUnconnected=off
  XMNSEH : Outport  Port=8  VectorParamsAs1DForOutWhenUnconnected=off
  G_NEW : Outport  Port=9  VectorParamsAs1DForOutWhenUnconnected=off
  wires:
  TESUB6 XMNSEB/2(G_NEW) -> TESUB6 XMNSEC/1(G)
  G/1 -> TESUB6 XMNSEA/1(G)
  TESUB6 XMNSEA/2(G_NEW) -> TESUB6 XMNSEB/1(G)
  TESUB6 XMNSEC/2(G_NEW) -> TESUB6 XMNSED/1(G)
  TESUB6 XMNSED/1(XMNSED) -> XMNSED/1  "XMNSED"
  TESUB6 XMNSEE/1(XMNSEE) -> XMNSEE/1  "XMNSEE"
  TESUB6 XMNSED/2(G_NEW) -> TESUB6 XMNSEE/1(G)
  TESUB6 XMNSEC/1(XMNSEC) -> XMNSEC/1  "XMNSEC"
  TESUB6 XMNSEA/1(XMNSEA) -> XMNSEA/1  "XMNSEA"
  TESUB6 XMNSEB/1(XMNSEB) -> XMNSEB/1  "XMNSEB"
  TESUB6 XMNSEE/2(G_NEW) -> TESUB6 XMNSEF/1(G)
  TESUB6 XMNSEF/2(G_NEW) -> TESUB6 XMNSEG/1(G)
  TESUB6 XMNSEG/2(G_NEW) -> TESUB6 XMNSEH/1(G)
  TESUB6 XMNSEH/2(G_NEW) -> G_NEW/1
  TESUB6 XMNSEF/1(XMNSEF) -> XMNSEF/1  "XMNSEF"
  TESUB6 XMNSEG/1(XMNSEG) -> XMNSEG/1  "XMNSEG"
  TESUB6 XMNSEH/1(XMNSEH) -> XMNSEH/1  "XMNSEH"

== system COSTEP/Random number generator/Stream Measurements SMEAS Gas analysis1/If Action Subsystem3/Subsystem/Stream 13/Subsystem ==
  G : Inport
  TESUB6 XMNSEA : Subsystem
  TESUB6 XMNSEB : Subsystem
  TESUB6 XMNSEC : Subsystem
  TESUB6 XMNSED : Subsystem
  TESUB6 XMNSEE : Subsystem
  TESUB6 XMNSEF : Subsystem
  TESUB6 XMNSEG : Subsystem
  TESUB6 XMNSEH : Subsystem
  XMNSEA : Outport  VectorParamsAs1DForOutWhenUnconnected=off
  XMNSEB : Outport  Port=2  VectorParamsAs1DForOutWhenUnconnected=off
  XMNSEC : Outport  Port=3  VectorParamsAs1DForOutWhenUnconnected=off
  XMNSED : Outport  Port=4  VectorParamsAs1DForOutWhenUnconnected=off
  XMNSEE : Outport  Port=5  VectorParamsAs1DForOutWhenUnconnected=off
  XMNSEF : Outport  Port=6  VectorParamsAs1DForOutWhenUnconnected=off
  XMNSEG : Outport  Port=7  VectorParamsAs1DForOutWhenUnconnected=off
  XMNSEH : Outport  Port=8  VectorParamsAs1DForOutWhenUnconnected=off
  G_NEW : Outport  Port=9  VectorParamsAs1DForOutWhenUnconnected=off
  wires:
  TESUB6 XMNSEB/2(G_NEW) -> TESUB6 XMNSEC/1(G)
  G/1 -> TESUB6 XMNSEA/1(G)
  TESUB6 XMNSEA/2(G_NEW) -> TESUB6 XMNSEB/1(G)
  TESUB6 XMNSEC/2(G_NEW) -> TESUB6 XMNSED/1(G)
  TESUB6 XMNSED/1(XMNSED) -> XMNSED/1  "XMNSED"
  TESUB6 XMNSEE/1(XMNSEE) -> XMNSEE/1  "XMNSEE"
  TESUB6 XMNSED/2(G_NEW) -> TESUB6 XMNSEE/1(G)
  TESUB6 XMNSEC/1(XMNSEC) -> XMNSEC/1  "XMNSEC"
  TESUB6 XMNSEA/1(XMNSEA) -> XMNSEA/1  "XMNSEA"
  TESUB6 XMNSEB/1(XMNSEB) -> XMNSEB/1  "XMNSEB"
  TESUB6 XMNSEE/2(G_NEW) -> TESUB6 XMNSEF/1(G)
  TESUB6 XMNSEF/2(G_NEW) -> TESUB6 XMNSEG/1(G)
  TESUB6 XMNSEG/2(G_NEW) -> TESUB6 XMNSEH/1(G)
  TESUB6 XMNSEH/2(G_NEW) -> G_NEW/1
  TESUB6 XMNSEF/1(XMNSEF) -> XMNSEF/1  "XMNSEF"
  TESUB6 XMNSEG/1(XMNSEG) -> XMNSEG/1  "XMNSEG"
  TESUB6 XMNSEH/1(XMNSEH) -> XMNSEH/1  "XMNSEH"

== system COSTEP/Random number generator/Stream Measurements SMEAS Gas analysis1/If Action Subsystem3/Subsystem/Stream 2/Subsystem ==
  G : Inport
  TESUB6 XMNSEA : Subsystem
  TESUB6 XMNSEB : Subsystem
  TESUB6 XMNSEC : Subsystem
  TESUB6 XMNSED : Subsystem
  TESUB6 XMNSEE : Subsystem
  TESUB6 XMNSEF : Subsystem
  TESUB6 XMNSEG : Subsystem
  TESUB6 XMNSEH : Subsystem
  XMNSEA : Outport  VectorParamsAs1DForOutWhenUnconnected=off
  XMNSEB : Outport  Port=2  VectorParamsAs1DForOutWhenUnconnected=off
  XMNSEC : Outport  Port=3  VectorParamsAs1DForOutWhenUnconnected=off
  XMNSED : Outport  Port=4  VectorParamsAs1DForOutWhenUnconnected=off
  XMNSEE : Outport  Port=5  VectorParamsAs1DForOutWhenUnconnected=off
  XMNSEF : Outport  Port=6  VectorParamsAs1DForOutWhenUnconnected=off
  XMNSEG : Outport  Port=7  VectorParamsAs1DForOutWhenUnconnected=off
  XMNSEH : Outport  Port=8  VectorParamsAs1DForOutWhenUnconnected=off
  G_NEW : Outport  Port=9  VectorParamsAs1DForOutWhenUnconnected=off
  wires:
  TESUB6 XMNSEB/2(G_NEW) -> TESUB6 XMNSEC/1(G)
  G/1 -> TESUB6 XMNSEA/1(G)
  TESUB6 XMNSEA/2(G_NEW) -> TESUB6 XMNSEB/1(G)
  TESUB6 XMNSEC/2(G_NEW) -> TESUB6 XMNSED/1(G)
  TESUB6 XMNSED/1(XMNSED) -> XMNSED/1  "XMNSED"
  TESUB6 XMNSEE/1(XMNSEE) -> XMNSEE/1  "XMNSEE"
  TESUB6 XMNSED/2(G_NEW) -> TESUB6 XMNSEE/1(G)
  TESUB6 XMNSEC/1(XMNSEC) -> XMNSEC/1  "XMNSEC"
  TESUB6 XMNSEA/1(XMNSEA) -> XMNSEA/1  "XMNSEA"
  TESUB6 XMNSEB/1(XMNSEB) -> XMNSEB/1  "XMNSEB"
  TESUB6 XMNSEE/2(G_NEW) -> TESUB6 XMNSEF/1(G)
  TESUB6 XMNSEF/2(G_NEW) -> TESUB6 XMNSEG/1(G)
  TESUB6 XMNSEG/2(G_NEW) -> TESUB6 XMNSEH/1(G)
  TESUB6 XMNSEH/2(G_NEW) -> G_NEW/1
  TESUB6 XMNSEF/1(XMNSEF) -> XMNSEF/1  "XMNSEF"
  TESUB6 XMNSEG/1(XMNSEG) -> XMNSEG/1  "XMNSEG"
  TESUB6 XMNSEH/1(XMNSEH) -> XMNSEH/1  "XMNSEH"

== system COSTEP/Random number generator/Stream Measurements SMEAS Gas analysis1/If Action Subsystem3/Subsystem/Stream 3/Subsystem ==
  G : Inport
  TESUB6 XMNSEA : Subsystem
  TESUB6 XMNSEB : Subsystem
  TESUB6 XMNSEC : Subsystem
  TESUB6 XMNSED : Subsystem
  TESUB6 XMNSEE : Subsystem
  TESUB6 XMNSEF : Subsystem
  TESUB6 XMNSEG : Subsystem
  TESUB6 XMNSEH : Subsystem
  XMNSEA : Outport  VectorParamsAs1DForOutWhenUnconnected=off
  XMNSEB : Outport  Port=2  VectorParamsAs1DForOutWhenUnconnected=off
  XMNSEC : Outport  Port=3  VectorParamsAs1DForOutWhenUnconnected=off
  XMNSED : Outport  Port=4  VectorParamsAs1DForOutWhenUnconnected=off
  XMNSEE : Outport  Port=5  VectorParamsAs1DForOutWhenUnconnected=off
  XMNSEF : Outport  Port=6  VectorParamsAs1DForOutWhenUnconnected=off
  XMNSEG : Outport  Port=7  VectorParamsAs1DForOutWhenUnconnected=off
  XMNSEH : Outport  Port=8  VectorParamsAs1DForOutWhenUnconnected=off
  G_NEW : Outport  Port=9  VectorParamsAs1DForOutWhenUnconnected=off
  wires:
  TESUB6 XMNSEB/2(G_NEW) -> TESUB6 XMNSEC/1(G)
  G/1 -> TESUB6 XMNSEA/1(G)
  TESUB6 XMNSEA/2(G_NEW) -> TESUB6 XMNSEB/1(G)
  TESUB6 XMNSEC/2(G_NEW) -> TESUB6 XMNSED/1(G)
  TESUB6 XMNSED/1(XMNSED) -> XMNSED/1  "XMNSED"
  TESUB6 XMNSEE/1(XMNSEE) -> XMNSEE/1  "XMNSEE"
  TESUB6 XMNSED/2(G_NEW) -> TESUB6 XMNSEE/1(G)
  TESUB6 XMNSEC/1(XMNSEC) -> XMNSEC/1  "XMNSEC"
  TESUB6 XMNSEA/1(XMNSEA) -> XMNSEA/1  "XMNSEA"
  TESUB6 XMNSEB/1(XMNSEB) -> XMNSEB/1  "XMNSEB"
  TESUB6 XMNSEE/2(G_NEW) -> TESUB6 XMNSEF/1(G)
  TESUB6 XMNSEF/2(G_NEW) -> TESUB6 XMNSEG/1(G)
  TESUB6 XMNSEG/2(G_NEW) -> TESUB6 XMNSEH/1(G)
  TESUB6 XMNSEH/2(G_NEW) -> G_NEW/1
  TESUB6 XMNSEF/1(XMNSEF) -> XMNSEF/1  "XMNSEF"
  TESUB6 XMNSEG/1(XMNSEG) -> XMNSEG/1  "XMNSEG"
  TESUB6 XMNSEH/1(XMNSEH) -> XMNSEH/1  "XMNSEH"

== system COSTEP/Random number generator/Stream Measurements SMEAS Gas analysis1/If Action Subsystem3/Subsystem/Stream 4/Subsystem ==
  G : Inport
  TESUB6 XMNSEA : Subsystem
  TESUB6 XMNSEB : Subsystem
  TESUB6 XMNSEC : Subsystem
  TESUB6 XMNSED : Subsystem
  TESUB6 XMNSEE : Subsystem
  TESUB6 XMNSEF : Subsystem
  TESUB6 XMNSEG : Subsystem
  TESUB6 XMNSEH : Subsystem
  XMNSEA : Outport  VectorParamsAs1DForOutWhenUnconnected=off
  XMNSEB : Outport  Port=2  VectorParamsAs1DForOutWhenUnconnected=off
  XMNSEC : Outport  Port=3  VectorParamsAs1DForOutWhenUnconnected=off
  XMNSED : Outport  Port=4  VectorParamsAs1DForOutWhenUnconnected=off
  XMNSEE : Outport  Port=5  VectorParamsAs1DForOutWhenUnconnected=off
  XMNSEF : Outport  Port=6  VectorParamsAs1DForOutWhenUnconnected=off
  XMNSEG : Outport  Port=7  VectorParamsAs1DForOutWhenUnconnected=off
  XMNSEH : Outport  Port=8  VectorParamsAs1DForOutWhenUnconnected=off
  G_NEW : Outport  Port=9  VectorParamsAs1DForOutWhenUnconnected=off
  wires:
  TESUB6 XMNSEB/2(G_NEW) -> TESUB6 XMNSEC/1(G)
  G/1 -> TESUB6 XMNSEA/1(G)
  TESUB6 XMNSEA/2(G_NEW) -> TESUB6 XMNSEB/1(G)
  TESUB6 XMNSEC/2(G_NEW) -> TESUB6 XMNSED/1(G)
  TESUB6 XMNSED/1(XMNSED) -> XMNSED/1  "XMNSED"
  TESUB6 XMNSEE/1(XMNSEE) -> XMNSEE/1  "XMNSEE"
  TESUB6 XMNSED/2(G_NEW) -> TESUB6 XMNSEE/1(G)
  TESUB6 XMNSEC/1(XMNSEC) -> XMNSEC/1  "XMNSEC"
  TESUB6 XMNSEA/1(XMNSEA) -> XMNSEA/1  "XMNSEA"
  TESUB6 XMNSEB/1(XMNSEB) -> XMNSEB/1  "XMNSEB"
  TESUB6 XMNSEE/2(G_NEW) -> TESUB6 XMNSEF/1(G)
  TESUB6 XMNSEF/2(G_NEW) -> TESUB6 XMNSEG/1(G)
  TESUB6 XMNSEG/2(G_NEW) -> TESUB6 XMNSEH/1(G)
  TESUB6 XMNSEH/2(G_NEW) -> G_NEW/1
  TESUB6 XMNSEF/1(XMNSEF) -> XMNSEF/1  "XMNSEF"
  TESUB6 XMNSEG/1(XMNSEG) -> XMNSEG/1  "XMNSEG"
  TESUB6 XMNSEH/1(XMNSEH) -> XMNSEH/1  "XMNSEH"

== system COSTEP/Random number generator/Stream Measurements SMEAS Gas analysis1/If Action Subsystem3/Subsystem/Stream 5/Subsystem ==
  G : Inport
  TESUB6 XMNSEA : Subsystem
  TESUB6 XMNSEB : Subsystem
  TESUB6 XMNSEC : Subsystem
  TESUB6 XMNSED : Subsystem
  TESUB6 XMNSEE : Subsystem
  TESUB6 XMNSEF : Subsystem
  TESUB6 XMNSEG : Subsystem
  TESUB6 XMNSEH : Subsystem
  XMNSEA : Outport  VectorParamsAs1DForOutWhenUnconnected=off
  XMNSEB : Outport  Port=2  VectorParamsAs1DForOutWhenUnconnected=off
  XMNSEC : Outport  Port=3  VectorParamsAs1DForOutWhenUnconnected=off
  XMNSED : Outport  Port=4  VectorParamsAs1DForOutWhenUnconnected=off
  XMNSEE : Outport  Port=5  VectorParamsAs1DForOutWhenUnconnected=off
  XMNSEF : Outport  Port=6  VectorParamsAs1DForOutWhenUnconnected=off
  XMNSEG : Outport  Port=7  VectorParamsAs1DForOutWhenUnconnected=off
  XMNSEH : Outport  Port=8  VectorParamsAs1DForOutWhenUnconnected=off
  G_NEW : Outport  Port=9  VectorParamsAs1DForOutWhenUnconnected=off
  wires:
  TESUB6 XMNSEB/2(G_NEW) -> TESUB6 XMNSEC/1(G)
  G/1 -> TESUB6 XMNSEA/1(G)
  TESUB6 XMNSEA/2(G_NEW) -> TESUB6 XMNSEB/1(G)
  TESUB6 XMNSEC/2(G_NEW) -> TESUB6 XMNSED/1(G)
  TESUB6 XMNSED/1(XMNSED) -> XMNSED/1  "XMNSED"
  TESUB6 XMNSEE/1(XMNSEE) -> XMNSEE/1  "XMNSEE"
  TESUB6 XMNSED/2(G_NEW) -> TESUB6 XMNSEE/1(G)
  TESUB6 XMNSEC/1(XMNSEC) -> XMNSEC/1  "XMNSEC"
  TESUB6 XMNSEA/1(XMNSEA) -> XMNSEA/1  "XMNSEA"
  TESUB6 XMNSEB/1(XMNSEB) -> XMNSEB/1  "XMNSEB"
  TESUB6 XMNSEE/2(G_NEW) -> TESUB6 XMNSEF/1(G)
  TESUB6 XMNSEF/2(G_NEW) -> TESUB6 XMNSEG/1(G)
  TESUB6 XMNSEG/2(G_NEW) -> TESUB6 XMNSEH/1(G)
  TESUB6 XMNSEH/2(G_NEW) -> G_NEW/1
  TESUB6 XMNSEF/1(XMNSEF) -> XMNSEF/1  "XMNSEF"
  TESUB6 XMNSEG/1(XMNSEG) -> XMNSEG/1  "XMNSEG"
  TESUB6 XMNSEH/1(XMNSEH) -> XMNSEH/1  "XMNSEH"

== system COSTEP/Random number generator/Stream Measurements SMEAS Gas analysis1/If Action Subsystem3/Subsystem/Stream 6/Subsystem ==
  G : Inport
  TESUB6 XMNSEA : Subsystem
  TESUB6 XMNSEB : Subsystem
  TESUB6 XMNSEC : Subsystem
  TESUB6 XMNSED : Subsystem
  TESUB6 XMNSEE : Subsystem
  TESUB6 XMNSEF : Subsystem
  TESUB6 XMNSEG : Subsystem
  TESUB6 XMNSEH : Subsystem
  XMNSEA : Outport  VectorParamsAs1DForOutWhenUnconnected=off
  XMNSEB : Outport  Port=2  VectorParamsAs1DForOutWhenUnconnected=off
  XMNSEC : Outport  Port=3  VectorParamsAs1DForOutWhenUnconnected=off
  XMNSED : Outport  Port=4  VectorParamsAs1DForOutWhenUnconnected=off
  XMNSEE : Outport  Port=5  VectorParamsAs1DForOutWhenUnconnected=off
  XMNSEF : Outport  Port=6  VectorParamsAs1DForOutWhenUnconnected=off
  XMNSEG : Outport  Port=7  VectorParamsAs1DForOutWhenUnconnected=off
  XMNSEH : Outport  Port=8  VectorParamsAs1DForOutWhenUnconnected=off
  G_NEW : Outport  Port=9  VectorParamsAs1DForOutWhenUnconnected=off
  wires:
  TESUB6 XMNSEB/2(G_NEW) -> TESUB6 XMNSEC/1(G)
  G/1 -> TESUB6 XMNSEA/1(G)
  TESUB6 XMNSEA/2(G_NEW) -> TESUB6 XMNSEB/1(G)
  TESUB6 XMNSEC/2(G_NEW) -> TESUB6 XMNSED/1(G)
  TESUB6 XMNSED/1(XMNSED) -> XMNSED/1  "XMNSED"
  TESUB6 XMNSEE/1(XMNSEE) -> XMNSEE/1  "XMNSEE"
  TESUB6 XMNSED/2(G_NEW) -> TESUB6 XMNSEE/1(G)
  TESUB6 XMNSEC/1(XMNSEC) -> XMNSEC/1  "XMNSEC"
  TESUB6 XMNSEA/1(XMNSEA) -> XMNSEA/1  "XMNSEA"
  TESUB6 XMNSEB/1(XMNSEB) -> XMNSEB/1  "XMNSEB"
  TESUB6 XMNSEE/2(G_NEW) -> TESUB6 XMNSEF/1(G)
  TESUB6 XMNSEF/2(G_NEW) -> TESUB6 XMNSEG/1(G)
  TESUB6 XMNSEG/2(G_NEW) -> TESUB6 XMNSEH/1(G)
  TESUB6 XMNSEH/2(G_NEW) -> G_NEW/1
  TESUB6 XMNSEF/1(XMNSEF) -> XMNSEF/1  "XMNSEF"
  TESUB6 XMNSEG/1(XMNSEG) -> XMNSEG/1  "XMNSEG"
  TESUB6 XMNSEH/1(XMNSEH) -> XMNSEH/1  "XMNSEH"

== system COSTEP/Random number generator/Stream Measurements SMEAS Gas analysis1/If Action Subsystem3/Subsystem/Stream 8/Subsystem ==
  G : Inport
  TESUB6 XMNSEA : Subsystem
  TESUB6 XMNSEB : Subsystem
  TESUB6 XMNSEC : Subsystem
  TESUB6 XMNSED : Subsystem
  TESUB6 XMNSEE : Subsystem
  TESUB6 XMNSEF : Subsystem
  TESUB6 XMNSEG : Subsystem
  TESUB6 XMNSEH : Subsystem
  XMNSEA : Outport  VectorParamsAs1DForOutWhenUnconnected=off
  XMNSEB : Outport  Port=2  VectorParamsAs1DForOutWhenUnconnected=off
  XMNSEC : Outport  Port=3  VectorParamsAs1DForOutWhenUnconnected=off
  XMNSED : Outport  Port=4  VectorParamsAs1DForOutWhenUnconnected=off
  XMNSEE : Outport  Port=5  VectorParamsAs1DForOutWhenUnconnected=off
  XMNSEF : Outport  Port=6  VectorParamsAs1DForOutWhenUnconnected=off
  XMNSEG : Outport  Port=7  VectorParamsAs1DForOutWhenUnconnected=off
  XMNSEH : Outport  Port=8  VectorParamsAs1DForOutWhenUnconnected=off
  G_NEW : Outport  Port=9  VectorParamsAs1DForOutWhenUnconnected=off
  wires:
  TESUB6 XMNSEB/2(G_NEW) -> TESUB6 XMNSEC/1(G)
  G/1 -> TESUB6 XMNSEA/1(G)
  TESUB6 XMNSEA/2(G_NEW) -> TESUB6 XMNSEB/1(G)
  TESUB6 XMNSEC/2(G_NEW) -> TESUB6 XMNSED/1(G)
  TESUB6 XMNSED/1(XMNSED) -> XMNSED/1  "XMNSED"
  TESUB6 XMNSEE/1(XMNSEE) -> XMNSEE/1  "XMNSEE"
  TESUB6 XMNSED/2(G_NEW) -> TESUB6 XMNSEE/1(G)
  TESUB6 XMNSEC/1(XMNSEC) -> XMNSEC/1  "XMNSEC"
  TESUB6 XMNSEA/1(XMNSEA) -> XMNSEA/1  "XMNSEA"
  TESUB6 XMNSEB/1(XMNSEB) -> XMNSEB/1  "XMNSEB"
  TESUB6 XMNSEE/2(G_NEW) -> TESUB6 XMNSEF/1(G)
  TESUB6 XMNSEF/2(G_NEW) -> TESUB6 XMNSEG/1(G)
  TESUB6 XMNSEG/2(G_NEW) -> TESUB6 XMNSEH/1(G)
  TESUB6 XMNSEH/2(G_NEW) -> G_NEW/1
  TESUB6 XMNSEF/1(XMNSEF) -> XMNSEF/1  "XMNSEF"
  TESUB6 XMNSEG/1(XMNSEG) -> XMNSEG/1  "XMNSEG"
  TESUB6 XMNSEH/1(XMNSEH) -> XMNSEH/1  "XMNSEH"
